simulink library "Prop_demo"  (R2025b)
settings: Solver=VariableStepAuto  StartTime=0.0  StopTime=10.0  RelTol=1e-3
undefined symbols (not defined in the file): cfd2d_ja, cfd2d_jl, cfd2d_kQ, cfd2d_kT, cfd2d_P1_CEF_X, cfd2d_P1_CEF_Y, cfd2d_P1_CEF_Z, cfd2d_P1_CEM_X, cfd2d_P1_CEM_Y, cfd2d_P1_CEM_Z, cfd2d_P5_CEF_X, cfd2d_P5_CEF_Y, cfd2d_P5_CEF_Z, cfd2d_P5_CEM_X, cfd2d_P5_CEM_Y, cfd2d_P5_CEM_Z, cfd3d_ja, cfd3d_jl, cfd3d_P2_CEF_X, cfd3d_P2_CEF_Y, cfd3d_P2_CEF_Z, cfd3d_P2_CEM_X, cfd3d_P2_CEM_Y, cfd3d_P2_CEM_Z, cfd3d_P6_CEF_X, cfd3d_P6_CEF_Y, cfd3d_P6_CEF_Z, cfd3d_P6_CEM_X, cfd3d_P6_CEM_Y, cfd3d_P6_CEM_Z, cfd3d_pitch, CoefBus, DF3000_V2_Prop, magnitude, Prop1, Prop2
libraries: simulink_extras x22, matrix_library x12, sharedtransform x12, simulink x6, DF3000_V2_Common x4
(part 4 of 4)

== matlab function Prop_demo/Prop2/MATLAB Function2 ==
  data: propAbs input; a6 output; r_self6 output; r_cross6 output; V input; Alpha_abs_local input; Pitch input; b6 output; CoefBus input
function [a6, r_self6, r_cross6, b6] = CoefQuery_DF3000_Bus(propAbs, V, Alpha_abs_local, Pitch, CoefBus)
%#codegen
% Inputs:
%   propAbs          : prop index (1..8)
%   V                : airspeed
%   Alpha_abs_local  : if hover -> Alpha ; if tilt -> Nac
%   Pitch            : tilt pitch (only used for tilt)
%   CoefBus          : Bus: CoefBusObj (from DF3000_CoefBus.mat)
%
% Outputs (6x1):
%   a6      : [Fx Fy Fz Mx My Mz]^T   (base coefficient a)
%   b6      : [Fx Fy Fz Mx My Mz]^T   (offset coefficient b)
%   r_self6 : same order, interpolated r
%   r_cross6: reserved (no rpm-diff data), zeros

a6       = zeros(6,1);
b6       = zeros(6,1);
r_self6  = ones (6,1);
r_cross6 = zeros(6,1);

p = int32(propAbs);
if p < 1 || p > 8
    return;
end

% classify
isTilt  = (p==2) || (p==3) || (p==6) || (p==7);
isHover = (p==1) || (p==4) || (p==5) || (p==8);

% mirror sign: Fy, Mx, Mz flip
sgnFy = 1.0; sgnMx = 1.0; sgnMz = 1.0;
if (p==3) || (p==4) || (p==7) || (p==8)
    sgnFy = -1.0; sgnMx = -1.0; sgnMz = -1.0;
end

if isTilt
    % Alpha_abs_local is Nac for tilt
    Nac = Alpha_abs_local;

    % base index: (2,3)->Prop2 ; (6,7)->Prop6
    baseK = int32(1);
    if (p==6) || (p==7)
        baseK = int32(2);
    end

    bpV = CoefBus.bpV_t;
    bpP = CoefBus.bpPitch_t;
    bpN = CoefBus.bpNac_t;

    % a
    aFx = interp3_trilin(bpV,bpP,bpN, CoefBus.aT_FX(:,:,:,baseK), V, Pitch, Nac);
    aFy = interp3_trilin(bpV,bpP,bpN, CoefBus.aT_FY(:,:,:,baseK), V, Pitch, Nac);
    aFz = interp3_trilin(bpV,bpP,bpN, CoefBus.aT_FZ(:,:,:,baseK), V, Pitch, Nac);
    aMx = interp3_trilin(bpV,bpP,bpN, CoefBus.aT_MX(:,:,:,baseK), V, Pitch, Nac);
    aMy = interp3_trilin(bpV,bpP,bpN, CoefBus.aT_MY(:,:,:,baseK), V, Pitch, Nac);
    aMz = interp3_trilin(bpV,bpP,bpN, CoefBus.aT_MZ(:,:,:,baseK), V, Pitch, Nac);

    % b
    bFx = interp3_trilin(bpV,bpP,bpN, CoefBus.bT_FX(:,:,:,baseK), V, Pitch, Nac);
    bFy = interp3_trilin(bpV,bpP,bpN, CoefBus.bT_FY(:,:,:,baseK), V, Pitch, Nac);
    bFz = interp3_trilin(bpV,bpP,bpN, CoefBus.bT_FZ(:,:,:,baseK), V, Pitch, Nac);
    bMx = interp3_trilin(bpV,bpP,bpN, CoefBus.bT_MX(:,:,:,baseK), V, Pitch, Nac);
    bMy = interp3_trilin(bpV,bpP,bpN, CoefBus.bT_MY(:,:,:,baseK), V, Pitch, Nac);
    bMz = interp3_trilin(bpV,bpP,bpN, CoefBus.bT_MZ(:,:,:,baseK), V, Pitch, Nac);

else
    % hover: Alpha_abs_local is Alpha
    Alpha = Alpha_abs_local;

    % base index: (1,4)->Prop1 ; (5,8)->Prop5
    baseK = int32(1);
    if (p==5) || (p==8)
        baseK = int32(2);
    end

    bpV = CoefBus.bpV_h;
    bpA = CoefBus.bpA_h;

    aFx = interp2_bilin(bpV,bpA, CoefBus.aH_FX(:,:,baseK), V, Alpha);
    aFy = interp2_bilin(bpV,bpA, CoefBus.aH_FY(:,:,baseK), V, Alpha);
    aFz = interp2_bilin(bpV,bpA, CoefBus.aH_FZ(:,:,baseK), V, Alpha);
    aMx = interp2_bilin(bpV,bpA, CoefBus.aH_MX(:,:,baseK), V, Alpha);
    aMy = interp2_bilin(bpV,bpA, CoefBus.aH_MY(:,:,baseK), V, Alpha);
    aMz = interp2_bilin(bpV,bpA, CoefBus.aH_MZ(:,:,baseK), V, Alpha);

    bFx = interp2_bilin(bpV,bpA, CoefBus.bH_FX(:,:,baseK), V, Alpha);
    bFy = interp2_bilin(bpV,bpA, CoefBus.bH_FY(:,:,baseK), V, Alpha);
    bFz = interp2_bilin(bpV,bpA, CoefBus.bH_FZ(:,:,baseK), V, Alpha);
    bMx = interp2_bilin(bpV,bpA, CoefBus.bH_MX(:,:,baseK), V, Alpha);
    bMy = interp2_bilin(bpV,bpA, CoefBus.bH_MY(:,:,baseK), V, Alpha);
    bMz = interp2_bilin(bpV,bpA, CoefBus.bH_MZ(:,:,baseK), V, Alpha);
end

% apply mirror sign to Fy, Mx, Mz (a/b/r 都一致处理)
a6(1)=aFx;
a6(2)=sgnFy*aFy;
a6(3)=aFz;
a6(4)=sgnMx*aMx;
a6(5)=aMy;
a6(6)=sgnMz*aMz;

b6(1)=bFx;
b6(2)=sgnFy*bFy;
b6(3)=bFz;
b6(4)=sgnMx*bMx;
b6(5)=bMy;
b6(6)=sgnMz*bMz;

end

%% ================= helpers (codegen-friendly) =================

function z = interp2_bilin(x,y,F,xq,yq)
x=double(x(:)); y=double(y(:)); F=double(F);
xq=double(xq); yq=double(yq);
nV=numel(x); nA=numel(y);
if nV<2||nA<2, z=F(1,1); return; end

% clamp interval search
if xq<=x(1), i=1; elseif xq>=x(nV), i=nV-1;
else
    i=1; while i<nV && xq>x(i+1), i=i+1; end
    if i>=nV, i=nV-1; end
end
if yq<=y(1), j=1; elseif yq>=y(nA), j=nA-1;
else
    j=1; while j<nA && yq>y(j+1), j=j+1; end
    if j>=nA, j=nA-1; end
end

tx=0; if x(i+1)>x(i), tx=(xq-x(i))/(x(i+1)-x(i)); end
ty=0; if y(j+1)>y(j), ty=(yq-y(j))/(y(j+1)-y(j)); end

F11=F(i,j);   F12=F(i,j+1);
F21=F(i+1,j); F22=F(i+1,j+1);

z=(1-tx)*((1-ty)*F11+ty*F12)+tx*((1-ty)*F21+ty*F22);
end

function v = interp3_trilin(x,y,z,F,xq,yq,zq)
% x: bpV, y: bpPitch, z: bpNac
x=double(x(:)); y=double(y(:)); z=double(z(:));
F=double(F);
xq=double(xq); yq=double(yq); zq=double(zq);

nx=numel(x); ny=numel(y); nz=numel(z);
if nx<2||ny<2||nz<2, v=F(1,1,1); return; end

% find i
if xq<=x(1), i=1; elseif xq>=x(nx), i=nx-1;
else
    i=1; while i<nx && xq>x(i+1), i=i+1; end
    if i>=nx, i=nx-1; end
end

% find j
if yq<=y(1), j=1; elseif yq>=y(ny), j=ny-1;
else
    j=1; while j<ny && yq>y(j+1), j=j+1; end
    if j>=ny, j=ny-1; end
end

% find k
if zq<=z(1), k=1; elseif zq>=z(nz), k=nz-1;
else
    k=1; while k<nz && zq>z(k+1), k=k+1; end
    if k>=nz, k=nz-1; end
end

tx=0; if x(i+1)>x(i), tx=(xq-x(i))/(x(i+1)-x(i)); end
ty=0; if y(j+1)>y(j), ty=(yq-y(j))/(y(j+1)-y(j)); end
tz=0; if z(k+1)>z(k), tz=(zq-z(k))/(z(k+1)-z(k)); end

% corners
c000 = F(i,  j,  k);
c010 = F(i,  j+1,k);
c100 = F(i+1,j,  k);
c110 = F(i+1,j+1,k);

c001 = F(i,  j,  k+1);
c011 = F(i,  j+1,k+1);
c101 = F(i+1,j,  k+1);
c111 = F(i+1,j+1,k+1);

c00 = (1-tx)*c000 + tx*c100;
c01 = (1-tx)*c001 + tx*c101;
c10 = (1-tx)*c010 + tx*c110;
c11 = (1-tx)*c011 + tx*c111;

c0 = (1-ty)*c00 + ty*c10;
c1 = (1-ty)*c01 + ty*c11;

v = (1-tz)*c0 + tz*c1;
end

== matlab function Prop_demo/Prop5/MATLAB Function ==
  data: u input; y output
function y = mate(u)

if u <= 4
    y = u+4;
else
    y = u-4;
end

== matlab function Prop_demo/Prop5/MATLAB Function2 ==
  data: propAbs input; a6 output; r_self6 output; r_cross6 output; V input; Alpha_abs_local input; RPM input; b6 output; CoefBus input
function [a6, r_self6, r_cross6, b6] = CoefQuery_DF3000_Bus( ...
    propAbs, V, Alpha_abs_local, RPM, CoefBus)
%#codegen
% Pitch is tilt-prop pitch for P2/P3/P6/P7 and actual RPM for hover props.
% The hover low-RPM branch returns direct load in b6 and zero a6.

a6       = zeros(6,1);
b6       = zeros(6,1);
r_self6  = ones(6,1);
r_cross6 = zeros(6,1);

p = int32(propAbs);
if p < 1 || p > 8
    return;
end

isTilt = (p==2) || (p==3) || (p==6) || (p==7);

sgnFy = 1.0;
sgnMx = 1.0;
sgnMz = 1.0;
if (p==3) || (p==4) || (p==7) || (p==8)
    sgnFy = -1.0;
    sgnMx = -1.0;
    sgnMz = -1.0;
end

if isTilt
    Nac = Alpha_abs_local;
    baseK = int32(1);
    if (p==6) || (p==7)
        baseK = int32(2);
    end

    bpV = CoefBus.bpV_t;
    bpP = CoefBus.bpPitch_t;
    bpN = CoefBus.bpNac_t;

    aFx = interp3_trilin(bpV,bpP,bpN, CoefBus.aT_FX(:,:,:,baseK), V, RPM, Nac);
    aFy = interp3_trilin(bpV,bpP,bpN, CoefBus.aT_FY(:,:,:,baseK), V, RPM, Nac);
    aFz = interp3_trilin(bpV,bpP,bpN, CoefBus.aT_FZ(:,:,:,baseK), V, RPM, Nac);
    aMx = interp3_trilin(bpV,bpP,bpN, CoefBus.aT_MX(:,:,:,baseK), V, RPM, Nac);
    aMy = interp3_trilin(bpV,bpP,bpN, CoefBus.aT_MY(:,:,:,baseK), V, RPM, Nac);
    aMz = interp3_trilin(bpV,bpP,bpN, CoefBus.aT_MZ(:,:,:,baseK), V, RPM, Nac);

    bFx = interp3_trilin(bpV,bpP,bpN, CoefBus.bT_FX(:,:,:,baseK), V, RPM, Nac);
    bFy = interp3_trilin(bpV,bpP,bpN, CoefBus.bT_FY(:,:,:,baseK), V, RPM, Nac);
    bFz = interp3_trilin(bpV,bpP,bpN, CoefBus.bT_FZ(:,:,:,baseK), V, RPM, Nac);
    bMx = interp3_trilin(bpV,bpP,bpN, CoefBus.bT_MX(:,:,:,baseK), V, RPM, Nac);
    bMy = interp3_trilin(bpV,bpP,bpN, CoefBus.bT_MY(:,:,:,baseK), V, RPM, Nac);
    bMz = interp3_trilin(bpV,bpP,bpN, CoefBus.bT_MZ(:,:,:,baseK), V, RPM, Nac);
else
    Alpha = Alpha_abs_local;
    RPM = max(double(RPM), 0.0);
    baseK = int32(1);
    if (p==5) || (p==8)
        baseK = int32(2);
    end

    bpV = CoefBus.bpV_h;
    bpA = CoefBus.bpA_h;
    rpmJoin = interp1_clamped(bpV, ...
        CoefBus.hoverLowRpmJoinRPM(:,baseK), V);
    useLowRpm = (CoefBus.hoverLowRpmEnable > 0.5) && (RPM < rpmJoin);

    if useLowRpm
        rpm2 = RPM * RPM;
        bpU = CoefBus.bpRPM2_h_low;
        aFx = 0.0; aFy = 0.0; aFz = 0.0;
        aMx = 0.0; aMy = 0.0; aMz = 0.0;
        bFx = interp3_trilin(bpV,bpA,bpU, CoefBus.lowH_FX(:,:,:,baseK), V, Alpha, rpm2);
        bFy = interp3_trilin(bpV,bpA,bpU, CoefBus.lowH_FY(:,:,:,baseK), V, Alpha, rpm2);
        bFz = interp3_trilin(bpV,bpA,bpU, CoefBus.lowH_FZ(:,:,:,baseK), V, Alpha, rpm2);
        bMx = interp3_trilin(bpV,bpA,bpU, CoefBus.lowH_MX(:,:,:,baseK), V, Alpha, rpm2);
        bMy = interp3_trilin(bpV,bpA,bpU, CoefBus.lowH_MY(:,:,:,baseK), V, Alpha, rpm2);
        bMz = interp3_trilin(bpV,bpA,bpU, CoefBus.lowH_MZ(:,:,:,baseK), V, Alpha, rpm2);
    else
        aFx = interp2_bilin(bpV,bpA, CoefBus.aH_FX(:,:,baseK), V, Alpha);
        aFy = interp2_bilin(bpV,bpA, CoefBus.aH_FY(:,:,baseK), V, Alpha);
        aFz = interp2_bilin(bpV,bpA, CoefBus.aH_FZ(:,:,baseK), V, Alpha);
        aMx = interp2_bilin(bpV,bpA, CoefBus.aH_MX(:,:,baseK), V, Alpha);
        aMy = interp2_bilin(bpV,bpA, CoefBus.aH_MY(:,:,baseK), V, Alpha);
        aMz = interp2_bilin(bpV,bpA, CoefBus.aH_MZ(:,:,baseK), V, Alpha);

        bFx = interp2_bilin(bpV,bpA, CoefBus.bH_FX(:,:,baseK), V, Alpha);
        bFy = interp2_bilin(bpV,bpA, CoefBus.bH_FY(:,:,baseK), V, Alpha);
        bFz = interp2_bilin(bpV,bpA, CoefBus.bH_FZ(:,:,baseK), V, Alpha);
        bMx = interp2_bilin(bpV,bpA, CoefBus.bH_MX(:,:,baseK), V, Alpha);
        bMy = interp2_bilin(bpV,bpA, CoefBus.bH_MY(:,:,baseK), V, Alpha);
        bMz = interp2_bilin(bpV,bpA, CoefBus.bH_MZ(:,:,baseK), V, Alpha);
    end
end

a6(1)=aFx;
a6(2)=sgnFy*aFy;
a6(3)=aFz;
a6(4)=sgnMx*aMx;
a6(5)=aMy;
a6(6)=sgnMz*aMz;

b6(1)=bFx;
b6(2)=sgnFy*bFy;
b6(3)=bFz;
b6(4)=sgnMx*bMx;
b6(5)=bMy;
b6(6)=sgnMz*bMz;
end

function z = interp1_clamped(x,F,xq)
x=double(x(:));
F=double(F(:));
xq=double(xq);
n=numel(x);
if n<2
    z=F(1);
    return;
end
if xq<=x(1)
    z=F(1);
    return;
elseif xq>=x(n)
    z=F(n);
    return;
end
i=1;
while i<n && xq>x(i+1)
    i=i+1;
end
if i>=n
    i=n-1;
end
t=0;
if x(i+1)>x(i)
    t=(xq-x(i))/(x(i+1)-x(i));
end
z=(1-t)*F(i)+t*F(i+1);
end

function z = interp2_bilin(x,y,F,xq,yq)
x=double(x(:));
y=double(y(:));
F=double(F);
xq=double(xq);
yq=double(yq);
nV=numel(x);
nA=numel(y);
if nV<2||nA<2
    z=F(1,1);
    return;
end
if xq<=x(1)
    i=1;
elseif xq>=x(nV)
    i=nV-1;
else
    i=1;
    while i<nV && xq>x(i+1)
        i=i+1;
    end
    if i>=nV
        i=nV-1;
    end
end
if yq<=y(1)
    j=1;
elseif yq>=y(nA)
    j=nA-1;
else
    j=1;
    while j<nA && yq>y(j+1)
        j=j+1;
    end
    if j>=nA
        j=nA-1;
    end
end
tx=0;
if x(i+1)>x(i)
    tx=(xq-x(i))/(x(i+1)-x(i));
end
ty=0;
if y(j+1)>y(j)
    ty=(yq-y(j))/(y(j+1)-y(j));
end
F11=F(i,j);
F12=F(i,j+1);
F21=F(i+1,j);
F22=F(i+1,j+1);
z=(1-tx)*((1-ty)*F11+ty*F12)+tx*((1-ty)*F21+ty*F22);
end

function v = interp3_trilin(x,y,z,F,xq,yq,zq)
x=double(x(:));
y=double(y(:));
z=double(z(:));
F=double(F);
xq=double(xq);
yq=double(yq);
zq=double(zq);
nx=numel(x);
ny=numel(y);
nz=numel(z);
if nx<2||ny<2||nz<2
    v=F(1,1,1);
    return;
end
if xq<=x(1)
    i=1;
elseif xq>=x(nx)
    i=nx-1;
else
    i=1;
    while i<nx && xq>x(i+1)
        i=i+1;
    end
    if i>=nx
        i=nx-1;
    end
end
if yq<=y(1)
    j=1;
elseif yq>=y(ny)
    j=ny-1;
else
    j=1;
    while j<ny && yq>y(j+1)
        j=j+1;
    end
    if j>=ny
        j=ny-1;
    end
end
if zq<=z(1)
    k=1;
elseif zq>=z(nz)
    k=nz-1;
else
    k=1;
    while k<nz && zq>z(k+1)
        k=k+1;
    end
    if k>=nz
        k=nz-1;
    end
end
tx=0;
if x(i+1)>x(i)
    tx=(xq-x(i))/(x(i+1)-x(i));
end
ty=0;
if y(j+1)>y(j)
    ty=(yq-y(j))/(y(j+1)-y(j));
end
tz=0;
if z(k+1)>z(k)
    tz=(zq-z(k))/(z(k+1)-z(k));
end
c000=F(i,j,k);
c010=F(i,j+1,k);
c100=F(i+1,j,k);
c110=F(i+1,j+1,k);
c001=F(i,j,k+1);
c011=F(i,j+1,k+1);
c101=F(i+1,j,k+1);
c111=F(i+1,j+1,k+1);
c00=(1-tx)*c000+tx*c100;
c01=(1-tx)*c001+tx*c101;
c10=(1-tx)*c010+tx*c110;
c11=(1-tx)*c011+tx*c111;
c0=(1-ty)*c00+ty*c10;
c1=(1-ty)*c01+ty*c11;
v=(1-tz)*c0+tz*c1;
end
